simulink model "cap_eq_circuit_pascal5_single_shot_stack"  (R2016b)
settings: Solver=FixedStepAuto  StartTime=0.0  StopTime=sim_time  FixedStep=sim_time*resolution  MinStep=0.001  RelTol=1e-4  EnableMultiTasking=on
values from neighbouring files (symbols this model uses):
  amps_in = double(amps_in)    [Sc.m]    (also in sc_model_single_shot_stack.m; test.m = 0; workspace_nedc_basic_sc.mat = 0; workspace_test_model.mat = 0)
undefined symbols (not defined in the file): capacitance, v_init1, v_init2
libraries: powerlib x360, simulink x8
(part 1 of 5)
settings Model: Creator=ttsh  LastModifiedBy=ttsh
settings SolverCC: ZeroCrossAlgorithm=Adaptive  AlgebraicLoopSolver=LineSearch  SolverResetMethod=Robust
settings DataIOCC: LimitDataPoints=on  SaveFormat=Array
settings OptimizationCC: LifeSpan=inf
settings DebuggingCC: SolverPrmCheckMsg=warning  AllowSymbolicDim=off  SFUnexpectedBacktrackingDiag=warning  SFNoUnconditionalDefaultTransitionDiag=warning  SFExecutionAtInitializationDiag=none
settings HardwareCC: ProdBitPerPointer=32  ProdBitPerSizeT=32  ProdBitPerPtrDiffT=32  ProdLargestAtomicFloat=None  ProdIntDivRoundTo=Undefined  ProdEndianess=Unspecified  ProdWordSize=32  ProdHWDeviceType=32-bit Generic
settings ModelReferenceCC: PropagateSignalLabelsOutOfModel=off
settings GRTTargetCC: TargetLangStandard=C89/C90 (ANSI)  GeneratePreprocessorConditionals=Disable all
settings ConfigComp: CovMetricSettings=dw  CovHtmlReporting=on  CovSaveCumulativeToWorkspaceVar=on  CovSaveSingleToWorkspaceVar=on  CovExternalEMLEnable=off  CovSFcnEnable=off

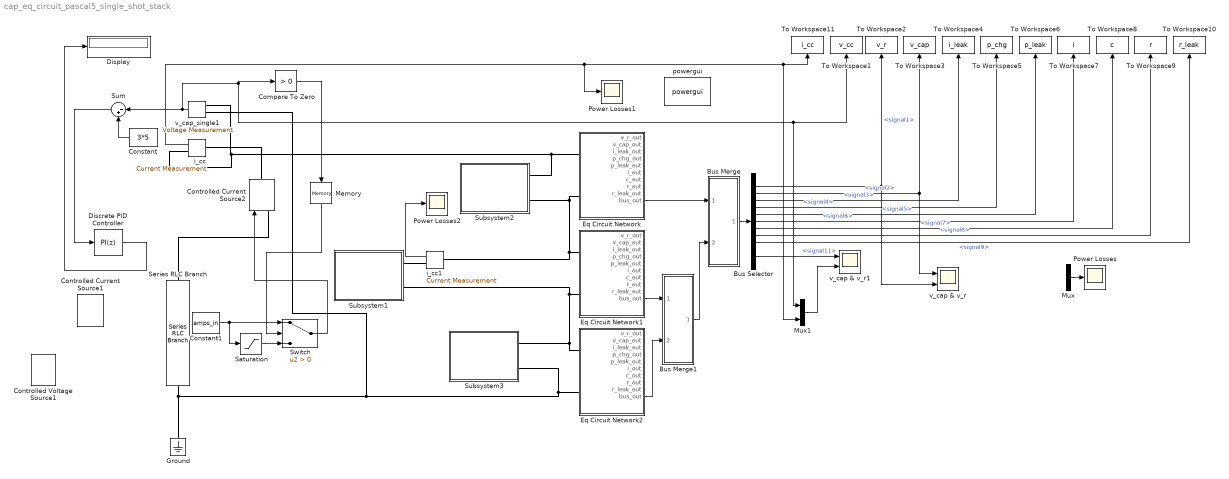
== system cap_eq_circuit_pascal5_single_shot_stack ==
  Bus Selector : BusSelector  OutputSignals=signal1,signal2,signal3,signal4,signal5,signal6,signal7,signal8,signal9,signal10,signal11
  Bus Merge : Subsystem
  Bus Merge1 : Subsystem
  Compare To Zero : simulink/Logic and Bit Operations/Compare To Zero  relop=>  OutDataTypeStr=boolean
  Constant : Constant  Value=3*5
  Constant1 : Constant  Value=amps_in
  Controlled Current Source1 : powerlib/Electrical Sources/Controlled Current Source  Initialize=on  Source_Type=DC  Amplitude=0  Phase=0  Frequency=0  Measurements=None
  Controlled Current Source2 : powerlib/Electrical Sources/Controlled Current Source  Initialize=on  Source_Type=DC  Amplitude=0  Phase=0  Frequency=0  Measurements=None
  Controlled Voltage Source1 : powerlib/Electrical Sources/Controlled Voltage Source  Initialize=on  Source_Type=DC  Amplitude=0  Phase=0  Frequency=0  Measurements=None
  Discrete PID Controller : simulink/Continuous/PID Controller  Controller=PI  TimeDomain=Discrete-time  SampleTime=-1  IntegratorMethod=Forward Euler  FilterMethod=Forward Euler  Form=Parallel  UseFilter=on  ControllerParametersSource=internal  P=1  I=0.02  D=0  N=100  InitialConditionSource=internal  InitialConditionForIntegrator=0  InitialConditionForFilter=0  ExternalReset=none  LimitOutput=on  UpperSaturationLimit=0.1  LowerSaturationLimit=0  LinearizeAsGain=off  AntiWindupMode=none  Kb=1  TrackingMode=off  Kt=1  PParamMin=[]  PParamMax=[]  IParamMin=[]  IParamMax=[]  DParamMin=[]  DParamMax=[]  NParamMin=[]  NParamMax=[]  KbParamMin=[]  KbParamMax=[]  KtParamMin=[]  KtParamMax=[]  POutMin=[]  POutMax=[]  IOutMin=[]  IOutMax=[]  DOutMin=[]  DOutMax=[]  NOutMin=[]  NOutMax=[]  KbOutMin=[]  KbOutMax=[]  KtOutMin=[]  KtOutMax=[]  IntegratorOutMin=[]  IntegratorOutMax=[]  FilterOutMin=[]  FilterOutMax=[]  SumOutMin=[]  SumOutMax=[]  SumI1OutMin=[]  SumI1OutMax=[]  SumI2OutMin=[]  SumI2OutMax=[]  SumI3OutMin=[]  SumI3OutMax=[]  SumDOutMin=[]  SumDOutMax=[]  SaturationOutMin=[]  SaturationOutMax=[]  IntegratorContinuousStateAttributes=''  IntegratorStateMustResolveToSignalObject=off  IntegratorRTWStateStorageClass=Auto  FilterContinuousStateAttributes=''  FilterStateMustResolveToSignalObject=off  FilterRTWStateStorageClass=Auto  DifferentiatorICPrevScaledInput=0  DifferentiatorOutMin=[]  DifferentiatorOutMax=[]
  Display : Display
  Eq Circuit Network : Subsystem  mask{r_leak=inf, c=capacitance, r_esr=0.01, ord=5, v_init1=v_init1(1), v_init2=v_init1(2), v_init3=v_init1(3), v_init4=v_init1(4), v_init5=v_init1(5)}
      mask prompts: r_leak "R Leak /ohm (inf for disabled)"; c "Capacitance /F"; r_esr "ESR"; ord "Elements (pascal order)"; v_init1 "Initial capacitor voltage"; v_init2 "Initial capacitor voltage"; v_init3 "Initial capacitor voltage"; v_init4 "Initial capacitor voltage"; v_init5 "Initial capacitor voltage"
  Eq Circuit Network1 : Subsystem  mask{r_leak=inf, c=capacitance, r_esr=0.01, ord=5, v_init1=v_init2(1), v_init2=v_init2(2), v_init3=v_init2(3), v_init4=v_init2(4), v_init5=v_init2(5)}
      mask prompts: r_leak "R Leak /ohm (inf for disabled)"; c "Capacitance /F"; r_esr "ESR"; ord "Elements (pascal order)"; v_init1 "Initial capacitor voltage"; v_init2 "Initial capacitor voltage"; v_init3 "Initial capacitor voltage"; v_init4 "Initial capacitor voltage"; v_init5 "Initial capacitor voltage"
  Eq Circuit Network2 : Subsystem  mask{r_leak=inf, c=capacitance, r_esr=0.01, ord=5, v_init1=v_init2(1), v_init2=v_init2(2), v_init3=v_init2(3), v_init4=v_init2(4), v_init5=v_init2(5)}
      mask prompts: r_leak "R Leak /ohm (inf for disabled)"; c "Capacitance /F"; r_esr "ESR"; ord "Elements (pascal order)"; v_init1 "Initial capacitor voltage"; v_init2 "Initial capacitor voltage"; v_init3 "Initial capacitor voltage"; v_init4 "Initial capacitor voltage"; v_init5 "Initial capacitor voltage"
  Ground : powerlib/Elements/Ground  LConnTagsString=a
  Memory : Memory  X0=1  InheritSampleTime=on
  Mux : Mux  Inputs=2
  Mux1 : Mux  Inputs=2
  Power Losses : Scope
  Power Losses1 : Scope
  Power Losses2 : Scope
  Saturation : Saturate  UpperLimit=inf  LowerLimit=0
  Series RLC Branch : powerlib/Elements/Series RLC Branch  LConnTagsString=__new0  RConnTagsString=__new0  BranchType=R  Resistance=0.1  Inductance=1e-9  SetiL0=off  InitialCurrent=0  Capacitance=1e-6  Setx0=off  InitialVoltage=0  Measurements=None
  Subsystem1 : Subsystem  mask{r=10, d=0.01, v_cut=5.1, v_min=0}
      mask prompts: r "Series resistance"; d "Rate limit"; v_cut "v cutoff"; v_min "v min"
  Subsystem2 : Subsystem  mask{r=10, d=0.01, v_cut=5.1, v_min=0}
      mask prompts: r "Series resistance"; d "Rate limit"; v_cut "v cutoff"; v_min "v min"
  Subsystem3 : Subsystem  mask{r=10, d=0.01, v_cut=5.1, v_min=0}
      mask prompts: r "Series resistance"; d "Rate limit"; v_cut "v cutoff"; v_min "v min"
  Sum : Sum  Inputs=|-+
  Switch : Switch  Criteria=u2 > Threshold
  To Workspace1 : ToWorkspace  VariableName=v_cc  SampleTime=-1
      settings: Save2DSignal=2-D array (concatenate along first dimension)
  To Workspace10 : ToWorkspace  VariableName=r_leak  SampleTime=-1
      settings: Save2DSignal=2-D array (concatenate along first dimension)
  To Workspace11 : ToWorkspace  VariableName=i_cc  SampleTime=-1
      settings: Save2DSignal=2-D array (concatenate along first dimension)
  To Workspace2 : ToWorkspace  VariableName=v_r  SampleTime=-1
      settings: Save2DSignal=2-D array (concatenate along first dimension)
  To Workspace3 : ToWorkspace  VariableName=v_cap  SampleTime=-1
      settings: Save2DSignal=2-D array (concatenate along first dimension)
  To Workspace4 : ToWorkspace  VariableName=i_leak  SampleTime=-1
      settings: Save2DSignal=2-D array (concatenate along first dimension)
  To Workspace5 : ToWorkspace  VariableName=p_chg  SampleTime=-1
      settings: Save2DSignal=2-D array (concatenate along first dimension)
  To Workspace6 : ToWorkspace  VariableName=p_leak  SampleTime=-1
      settings: Save2DSignal=2-D array (concatenate along first dimension)
  To Workspace7 : ToWorkspace  VariableName=i  SampleTime=-1
      settings: Save2DSignal=2-D array (concatenate along first dimension)
  To Workspace8 : ToWorkspace  VariableName=c  SampleTime=-1
      settings: Save2DSignal=2-D array (concatenate along first dimension)
  To Workspace9 : ToWorkspace  VariableName=r  SampleTime=-1
      settings: Save2DSignal=2-D array (concatenate along first dimension)
  i_cc : powerlib/Measurements/Current Measurement  PhasorSimulation=off  OutputType=Complex  PSBequivalent=0
  i_cc1 : powerlib/Measurements/Current Measurement  PhasorSimulation=off  OutputType=Complex  PSBequivalent=0
  powergui : powerlib/powergui  Priority=1  SimulationMode=Continuous  SolverType=Tustin  SampleTime=50e-6  frequency=60  SPID=on  DisableSnubberDevices=on  DisableRonSwitches=on  DisableVfSwitches=on  SwTol=0  DisplayEquations=off  Interpol=off  ExternalGateDelay=off  methode=off  Ts=0  FunctionMessages=off  echomessages=off  HookPort=off  EnableUseOfTLC=off  x0status=blocks  frequencyindice=0  Pbase=100e6  ErrMax=1e-4  Iterations=50  UnitsV=V  UnitsW=W  buscounter=0  RestoreLinks=warning  ResistiveCurrentMeasurement=off  Frange=[0:2:500]  Ylog=off  Xlog=on  ShowGrid=off  save=off  variable=ZData  structure=0  ZoomFFT=off  StartTime=0.0  cycles=1  DisplayStyle=1  fundamental=60  FreqAxis=off  MaxFrequency=1000  frequencyindicesteady=1  RmsSteady=1  display=off
  v_cap & v_r : Scope  NumInputPorts=2
  v_cap & v_r1 : Scope  NumInputPorts=2
  v_cap_single1 : powerlib/Measurements/Voltage Measurement  PhasorSimulation=off  OutputType=Complex  PSBequivalent=0
  wires:
  Mux/1 -> Power Losses/1
  i_cc/1 -> Power Losses1/1, Mux1/2, To Workspace11/1
  Eq Circuit Network/10(bus_out) -> Bus Merge/1(bus_1_in)
  Bus Merge/1(bus_out) -> Bus Selector/1
  Bus Selector/1 -> v_cap & v_r/2, To Workspace2/1  "<signal1>"
  Bus Selector/2 -> v_cap & v_r/1, To Workspace3/1  "<signal2>"
  Bus Selector/3 -> To Workspace4/1  "<signal3>"
  Bus Selector/4 -> To Workspace5/1  "<signal4>"
  Bus Selector/5 -> To Workspace6/1  "<signal5>"
  Bus Selector/6 -> To Workspace7/1  "<signal6>"
  Bus Selector/7 -> To Workspace8/1  "<signal7>"
  Bus Selector/8 -> To Workspace9/1  "<signal8>"
  Bus Selector/9 -> To Workspace10/1  "<signal9>"
  Bus Selector/11 -> v_cap & v_r1/1  "<signal11>"
  v_cap_single1/1 -> Sum/1, Compare To Zero/1, Mux1/1, To Workspace1/1
  Discrete PID Controller/1 -> Display/1
  Constant/1 -> Sum/2
  Sum/1 -> Discrete PID Controller/1
  Eq Circuit Network1/10(bus_out) -> Bus Merge1/1(bus_1_in)
  Eq Circuit Network2/10(bus_out) -> Bus Merge1/2(bus_2_in)
  Bus Merge1/1(bus_out) -> Bus Merge/2(bus_2_in)
  Mux1/1 -> v_cap & v_r1/2
  i_cc1/1 -> Power Losses2/1
  Constant1/1 -> Switch/1, Saturation/1
  Saturation/1 -> Switch/3
  Compare To Zero/1 -> Memory/1
  Switch/1 -> Controlled Current Source2/1
  Memory/1 -> Switch/2
  connections:
  v_cap_single1/LConn1 -- i_cc/RConn1 -- Subsystem2/RConn1 -- Eq Circuit Network/LConn1
  Eq Circuit Network/LConn2 -- Subsystem2/RConn2 -- i_cc1/LConn1 -- Eq Circuit Network1/LConn1
  Eq Circuit Network1/LConn2 -- Subsystem1/RConn2 -- Eq Circuit Network2/LConn1 -- Subsystem3/RConn1
  Controlled Current Source2/LConn1 -- Series RLC Branch/LConn1
  Controlled Current Source2/RConn1 -- i_cc/LConn1
  Series RLC Branch/RConn1 -- Ground/LConn1 -- v_cap_single1/LConn2 -- Eq Circuit Network2/LConn2 -- Subsystem3/RConn2
  Subsystem1/RConn1 -- i_cc1/RConn1

== system cap_eq_circuit_pascal5_single_shot_stack/Bus Merge ==
  bus_1_in : Inport
  bus_2_in : Inport  Port=2
  Bus Creator : BusCreator  Inputs=11
  Bus Selector : BusSelector  OutputSignals=signal1,signal2,signal3,signal4,signal5,signal6,signal7,signal8,signal9,signal10,signal11
  Bus Selector1 : BusSelector  OutputSignals=signal1,signal2,signal3,signal4,signal5,signal6,signal7,signal8,signal9,signal10,signal11
  Mux{1..11} (11 alike) : Mux  Inputs=2
  bus_out : Outport
  wires:
  bus_1_in/1 -> Bus Selector/1
  bus_2_in/1 -> Bus Selector1/1
  Bus Creator/1 -> bus_out/1
  Bus Selector/1 -> Mux1/1  "<signal1>"
  Bus Selector1/2 -> Mux2/2  "<signal2>"
  Bus Selector/3 -> Mux3/1  "<signal3>"
  Bus Selector1/4 -> Mux4/2  "<signal4>"
  Bus Selector/5 -> Mux5/1  "<signal5>"
  Bus Selector1/6 -> Mux6/1  "<signal6>"
  Bus Selector/7 -> Mux7/1  "<signal7>"
  Bus Selector1/8 -> Mux8/1  "<signal8>"
  Bus Selector1/10 -> Mux10/1  "<signal10>"
  Bus Selector/11 -> Mux11/1  "<signal11>"
  Bus Selector/9 -> Mux9/1  "<signal9>"
  Bus Selector/2 -> Mux2/1  "<signal2>"
  Bus Selector/4 -> Mux4/1  "<signal4>"
  Bus Selector/6 -> Mux6/2  "<signal6>"
  Bus Selector/8 -> Mux8/2  "<signal8>"
  Bus Selector/10 -> Mux10/2  "<signal10>"
  Bus Selector1/1 -> Mux1/2  "<signal1>"
  Bus Selector1/3 -> Mux3/2  "<signal3>"
  Bus Selector1/5 -> Mux5/2  "<signal5>"
  Bus Selector1/7 -> Mux7/2  "<signal7>"
  Bus Selector1/9 -> Mux9/2  "<signal9>"
  Bus Selector1/11 -> Mux11/2  "<signal11>"
  Mux1/1 -> Bus Creator/1
  Mux3/1 -> Bus Creator/3
  Mux5/1 -> Bus Creator/5
  Mux7/1 -> Bus Creator/7
  Mux9/1 -> Bus Creator/9
  Mux11/1 -> Bus Creator/11
  Mux2/1 -> Bus Creator/2
  Mux4/1 -> Bus Creator/4
  Mux6/1 -> Bus Creator/6
  Mux8/1 -> Bus Creator/8
  Mux10/1 -> Bus Creator/10

== system cap_eq_circuit_pascal5_single_shot_stack/Bus Merge1 ==
  bus_1_in : Inport
  bus_2_in : Inport  Port=2
  Bus Creator : BusCreator  Inputs=11
  Bus Selector : BusSelector  OutputSignals=signal1,signal2,signal3,signal4,signal5,signal6,signal7,signal8,signal9,signal10,signal11
  Bus Selector1 : BusSelector  OutputSignals=signal1,signal2,signal3,signal4,signal5,signal6,signal7,signal8,signal9,signal10,signal11
  Mux{1..11} (11 alike) : Mux  Inputs=2
  bus_out : Outport
  wires:
  Mux10/1 -> Bus Creator/10
  Mux8/1 -> Bus Creator/8
  Mux6/1 -> Bus Creator/6
  Mux4/1 -> Bus Creator/4
  Mux2/1 -> Bus Creator/2
  Mux11/1 -> Bus Creator/11
  Mux9/1 -> Bus Creator/9
  Mux7/1 -> Bus Creator/7
  Mux5/1 -> Bus Creator/5
  Mux3/1 -> Bus Creator/3
  Mux1/1 -> Bus Creator/1
  Bus Selector1/11 -> Mux11/2  "<signal11>"
  Bus Selector1/9 -> Mux9/2  "<signal9>"
  Bus Selector1/7 -> Mux7/2  "<signal7>"
  Bus Selector1/5 -> Mux5/2  "<signal5>"
  Bus Selector1/3 -> Mux3/2  "<signal3>"
  Bus Selector1/1 -> Mux1/2  "<signal1>"
  Bus Selector/10 -> Mux10/2  "<signal10>"
  Bus Selector/8 -> Mux8/2  "<signal8>"
  Bus Selector/6 -> Mux6/2  "<signal6>"
  Bus Selector/4 -> Mux4/1  "<signal4>"
  Bus Selector/2 -> Mux2/1  "<signal2>"
  Bus Selector/9 -> Mux9/1  "<signal9>"
  Bus Selector/11 -> Mux11/1  "<signal11>"
  Bus Selector1/10 -> Mux10/1  "<signal10>"
  Bus Selector1/8 -> Mux8/1  "<signal8>"
  Bus Selector/7 -> Mux7/1  "<signal7>"
  Bus Selector1/6 -> Mux6/1  "<signal6>"
  Bus Selector/5 -> Mux5/1  "<signal5>"
  Bus Selector1/4 -> Mux4/2  "<signal4>"
  Bus Selector/3 -> Mux3/1  "<signal3>"
  Bus Selector1/2 -> Mux2/2  "<signal2>"
  Bus Selector/1 -> Mux1/1  "<signal1>"
  Bus Creator/1 -> bus_out/1
  bus_2_in/1 -> Bus Selector1/1
  bus_1_in/1 -> Bus Selector/1

== system cap_eq_circuit_pascal5_single_shot_stack/Eq Circuit Network ==
  note: 6x 700R
  note: 4x 1k4
  note: 4x 625R
  note: 1x 550R
  note: 1x 4k
  Bus Creator : BusCreator  Inputs=11
  Subsystem : Subsystem  mask{c=c, r_esr=625, r_leak=r_leak, v_init=v_init2}
      mask prompts: c "Capacitance /F"; r_esr "Series resistance /ohm"; r_leak "Leak resistance /ohm (inf for disabled)"; v_init "Initial capacitor voltage"
  Subsystem1 : Subsystem  mask{c=c, r_esr=1.4e3, r_leak=r_leak, v_init=v_init4}
      mask prompts: c "Capacitance /F"; r_esr "Series resistance /ohm"; r_leak "Leak resistance /ohm (inf for disabled)"; v_init "Initial capacitor voltage"
  Subsystem2 : Subsystem  mask{c=c, r_esr=700, r_leak=r_leak, v_init=v_init3}
      mask prompts: c "Capacitance /F"; r_esr "Series resistance /ohm"; r_leak "Leak resistance /ohm (inf for disabled)"; v_init "Initial capacitor voltage"
  Subsystem5 : Subsystem  mask{c=c, r_esr=4e3, r_leak=r_leak, v_init=v_init5}
      mask prompts: c "Capacitance /F"; r_esr "Series resistance /ohm"; r_leak "Leakage resistance /ohm (inf for disabled)"; v_init "Initial capacitor voltage"
  Subsystem8 : Subsystem  mask{c=c, r_esr=550, r_leak=r_leak, v_init=v_init1}
      mask prompts: c "Capacitance /F"; r_esr "Series resistance /ohm"; r_leak "Leakage resistance /ohm (inf for disabled)"; v_init "Initial capacitor voltage"
  v_cap_single : powerlib/Measurements/Voltage Measurement  PhasorSimulation=off  OutputType=Complex  PSBequivalent=0
  VCC_in : PMIOPort  Port=1  Side=Left
  VSS_in : PMIOPort  Port=2  Side=Left
  VCC_out : PMIOPort  Port=3  Side=Right
  VSS_out : PMIOPort  Port=4  Side=Right
  v_r_out : Outport
  v_cap_out : Outport  Port=2
  i_leak_out : Outport  Port=3
  p_chg_out : Outport  Port=4
  p_leak_out : Outport  Port=5
  i_out : Outport  Port=6
  c_out : Outport  Port=7
  r_out : Outport  Port=8
  r_leak_out : Outport  Port=9
  bus_out : Outport  Port=10
  wires:
  Subsystem5/5(p_leak_out) -> Bus Creator/5, p_leak_out/1
  Subsystem5/6(i_out) -> Bus Creator/6, i_out/1
  Subsystem5/4(p_chg_out) -> Bus Creator/4, p_chg_out/1
  Subsystem5/7(c_out) -> Bus Creator/7, c_out/1
  Subsystem5/3(i_leak_out) -> Bus Creator/3, i_leak_out/1
  Subsystem5/8(r_out) -> Bus Creator/8, r_out/1
  Subsystem5/2(v_cap_out) -> Bus Creator/2, v_cap_out/1
  Subsystem5/9(r_leak_out) -> Bus Creator/9, r_leak_out/1
  Subsystem5/1(v_r_out) -> Bus Creator/1, v_r_out/1
  Subsystem8/3(i_leak_out) -> Subsystem/3(In3)
  Subsystem8/6(i_out) -> Subsystem/6(In6)
  Subsystem8/9(r_leak_out) -> Subsystem/9(In9)
  Subsystem8/4(p_chg_out) -> Subsystem/4(In4)
  Subsystem8/10(l_out) -> Subsystem/10(In10)
  Subsystem8/8(r_out) -> Subsystem/8(In8)
  Subsystem8/5(p_leak_out) -> Subsystem/5(In5)
  Subsystem8/7(c_out) -> Subsystem/7(In7)
  Subsystem8/1(v_r_out) -> Subsystem/1(In1)
  Subsystem8/2(v_cap_out) -> Subsystem/2(In2)
  Subsystem1/6(Out6) -> Subsystem5/6(i_in)
  Subsystem1/8(Out8) -> Subsystem5/8(r_in)
  Subsystem1/4(Out4) -> Subsystem5/4(p_chg_in)
  Subsystem1/7(Out7) -> Subsystem5/7(c_in)
  Subsystem1/9(Out9) -> Subsystem5/9(r_leak_in)
  Subsystem1/3(Out3) -> Subsystem5/3(i_leak_in)
  Subsystem1/10(Out10) -> Subsystem5/10(l_in)
  Subsystem1/5(Out5) -> Subsystem5/5(p_leak_in)
  Subsystem1/2(Out2) -> Subsystem5/2(v_cap_in)
  Subsystem1/1(Out1) -> Subsystem5/1(v_r_in)
  Subsystem/3(Out3) -> Subsystem2/3(In3)
  Subsystem/10(Out10) -> Subsystem2/10(In10)
  Subsystem/8(Out8) -> Subsystem2/8(In8)
  Subsystem/1(Out1) -> Subsystem2/1(In1)
  Subsystem/2(Out2) -> Subsystem2/2(In2)
  Subsystem/6(Out6) -> Subsystem2/6(In6)
  Subsystem/9(Out9) -> Subsystem2/9(In9)
  Subsystem/7(Out7) -> Subsystem2/7(In7)
  Subsystem/4(Out4) -> Subsystem2/4(In4)
  Subsystem/5(Out5) -> Subsystem2/5(In5)
  Subsystem2/5(Out5) -> Subsystem1/5(In5)
  Subsystem2/8(Out8) -> Subsystem1/8(In8)
  Subsystem2/6(Out6) -> Subsystem1/6(In6)
  Subsystem2/2(Out2) -> Subsystem1/2(In2)
  Subsystem2/10(Out10) -> Subsystem1/10(In10)
  Subsystem2/9(Out9) -> Subsystem1/9(In9)
  Subsystem2/1(Out1) -> Subsystem1/1(In1)
  Subsystem2/3(Out3) -> Subsystem1/3(In3)
  Subsystem2/4(Out4) -> Subsystem1/4(In4)
  Subsystem2/7(Out7) -> Subsystem1/7(In7)
  v_cap_single/1 -> Bus Creator/11
  Subsystem5/10(l_out) -> Bus Creator/10
  Bus Creator/1 -> bus_out/1
  connections:
  Subsystem8/LConn1 -- VCC_in/RConn1
  VSS_in/RConn1 -- Subsystem8/LConn2
  Subsystem8/RConn2 -- Subsystem/LConn2
  Subsystem8/RConn1 -- Subsystem/LConn1
  Subsystem1/RConn2 -- Subsystem5/LConn2
  Subsystem1/RConn1 -- Subsystem5/LConn1
  Subsystem/RConn1 -- Subsystem2/LConn1
  Subsystem/RConn2 -- Subsystem2/LConn2
  Subsystem1/LConn2 -- Subsystem2/RConn2
  Subsystem1/LConn1 -- Subsystem2/RConn1
  VCC_out/RConn1 -- v_cap_single/LConn1 -- Subsystem5/RConn1
  Subsystem5/RConn2 -- v_cap_single/LConn2 -- VSS_out/RConn1

== system cap_eq_circuit_pascal5_single_shot_stack/Eq Circuit Network1 ==
  note: 1x 4k
  note: 1x 550R
  note: 4x 625R
  note: 4x 1k4
  note: 6x 700R
  Bus Creator : BusCreator  Inputs=11
  Subsystem : Subsystem  mask{c=c, r_esr=625, r_leak=r_leak, v_init=v_init2}
      mask prompts: c "Capacitance /F"; r_esr "Series resistance /ohm"; r_leak "Leak resistance /ohm (inf for disabled)"; v_init "Initial capacitor voltage"
  Subsystem1 : Subsystem  mask{c=c, r_esr=1.4e3, r_leak=r_leak, v_init=v_init4}
      mask prompts: c "Capacitance /F"; r_esr "Series resistance /ohm"; r_leak "Leak resistance /ohm (inf for disabled)"; v_init "Initial capacitor voltage"
  Subsystem2 : Subsystem  mask{c=c, r_esr=700, r_leak=r_leak, v_init=v_init3}
      mask prompts: c "Capacitance /F"; r_esr "Series resistance /ohm"; r_leak "Leak resistance /ohm (inf for disabled)"; v_init "Initial capacitor voltage"
  Subsystem5 : Subsystem  mask{c=c, r_esr=4e3, r_leak=r_leak, v_init=v_init5}
      mask prompts: c "Capacitance /F"; r_esr "Series resistance /ohm"; r_leak "Leakage resistance /ohm (inf for disabled)"; v_init "Initial capacitor voltage"
  Subsystem8 : Subsystem  mask{c=c, r_esr=550, r_leak=r_leak, v_init=v_init1}
      mask prompts: c "Capacitance /F"; r_esr "Series resistance /ohm"; r_leak "Leakage resistance /ohm (inf for disabled)"; v_init "Initial capacitor voltage"
  v_cap_single : powerlib/Measurements/Voltage Measurement  PhasorSimulation=off  OutputType=Complex  PSBequivalent=0
  VCC_in : PMIOPort  Port=1  Side=Left
  VSS_in : PMIOPort  Port=2  Side=Left
  VCC_out : PMIOPort  Port=3  Side=Right
  VSS_out : PMIOPort  Port=4  Side=Right
  v_r_out : Outport
  v_cap_out : Outport  Port=2
  i_leak_out : Outport  Port=3
  p_chg_out : Outport  Port=4
  p_leak_out : Outport  Port=5
  i_out : Outport  Port=6
  c_out : Outport  Port=7
  r_out : Outport  Port=8
  r_leak_out : Outport  Port=9
  bus_out : Outport  Port=10
  wires:
  Bus Creator/1 -> bus_out/1
  Subsystem5/10(l_out) -> Bus Creator/10
  v_cap_single/1 -> Bus Creator/11
  Subsystem2/7(Out7) -> Subsystem1/7(In7)
  Subsystem2/4(Out4) -> Subsystem1/4(In4)
  Subsystem2/3(Out3) -> Subsystem1/3(In3)
  Subsystem2/1(Out1) -> Subsystem1/1(In1)
  Subsystem2/9(Out9) -> Subsystem1/9(In9)
  Subsystem2/10(Out10) -> Subsystem1/10(In10)
  Subsystem2/2(Out2) -> Subsystem1/2(In2)
  Subsystem2/6(Out6) -> Subsystem1/6(In6)
  Subsystem2/8(Out8) -> Subsystem1/8(In8)
  Subsystem2/5(Out5) -> Subsystem1/5(In5)
  Subsystem/5(Out5) -> Subsystem2/5(In5)
  Subsystem/4(Out4) -> Subsystem2/4(In4)
  Subsystem/7(Out7) -> Subsystem2/7(In7)
  Subsystem/9(Out9) -> Subsystem2/9(In9)
  Subsystem/6(Out6) -> Subsystem2/6(In6)
  Subsystem/2(Out2) -> Subsystem2/2(In2)
  Subsystem/1(Out1) -> Subsystem2/1(In1)
  Subsystem/8(Out8) -> Subsystem2/8(In8)
  Subsystem/10(Out10) -> Subsystem2/10(In10)
  Subsystem/3(Out3) -> Subsystem2/3(In3)
  Subsystem1/1(Out1) -> Subsystem5/1(v_r_in)
  Subsystem1/2(Out2) -> Subsystem5/2(v_cap_in)
  Subsystem1/5(Out5) -> Subsystem5/5(p_leak_in)
  Subsystem1/10(Out10) -> Subsystem5/10(l_in)
  Subsystem1/3(Out3) -> Subsystem5/3(i_leak_in)
  Subsystem1/9(Out9) -> Subsystem5/9(r_leak_in)
  Subsystem1/7(Out7) -> Subsystem5/7(c_in)
  Subsystem1/4(Out4) -> Subsystem5/4(p_chg_in)
  Subsystem1/8(Out8) -> Subsystem5/8(r_in)
  Subsystem1/6(Out6) -> Subsystem5/6(i_in)
  Subsystem8/2(v_cap_out) -> Subsystem/2(In2)
  Subsystem8/1(v_r_out) -> Subsystem/1(In1)
  Subsystem8/7(c_out) -> Subsystem/7(In7)
  Subsystem8/5(p_leak_out) -> Subsystem/5(In5)
  Subsystem8/8(r_out) -> Subsystem/8(In8)
  Subsystem8/10(l_out) -> Subsystem/10(In10)
  Subsystem8/4(p_chg_out) -> Subsystem/4(In4)
  Subsystem8/9(r_leak_out) -> Subsystem/9(In9)
  Subsystem8/6(i_out) -> Subsystem/6(In6)
  Subsystem8/3(i_leak_out) -> Subsystem/3(In3)
  Subsystem5/1(v_r_out) -> v_r_out/1, Bus Creator/1
  Subsystem5/9(r_leak_out) -> r_leak_out/1, Bus Creator/9
  Subsystem5/2(v_cap_out) -> v_cap_out/1, Bus Creator/2
  Subsystem5/8(r_out) -> r_out/1, Bus Creator/8
  Subsystem5/3(i_leak_out) -> i_leak_out/1, Bus Creator/3
  Subsystem5/7(c_out) -> c_out/1, Bus Creator/7
  Subsystem5/4(p_chg_out) -> p_chg_out/1, Bus Creator/4
  Subsystem5/6(i_out) -> i_out/1, Bus Creator/6
  Subsystem5/5(p_leak_out) -> p_leak_out/1, Bus Creator/5
  connections:
  v_cap_single/LConn2 -- Subsystem5/RConn2 -- VSS_out/RConn1
  v_cap_single/LConn1 -- VCC_out/RConn1 -- Subsystem5/RConn1
  Subsystem1/LConn1 -- Subsystem2/RConn1
  Subsystem1/LConn2 -- Subsystem2/RConn2
  Subsystem/RConn2 -- Subsystem2/LConn2
  Subsystem/RConn1 -- Subsystem2/LConn1
  Subsystem1/RConn1 -- Subsystem5/LConn1
  Subsystem1/RConn2 -- Subsystem5/LConn2
  Subsystem8/RConn1 -- Subsystem/LConn1
  Subsystem8/RConn2 -- Subsystem/LConn2
  VSS_in/RConn1 -- Subsystem8/LConn2
  Subsystem8/LConn1 -- VCC_in/RConn1

== system cap_eq_circuit_pascal5_single_shot_stack/Eq Circuit Network2 ==
  note: 6x 700R
  note: 4x 1k4
  note: 4x 625R
  note: 1x 550R
  note: 1x 4k
  Bus Creator : BusCreator  Inputs=11
  Subsystem : Subsystem  mask{c=c, r_esr=625, r_leak=r_leak, v_init=v_init2}
      mask prompts: c "Capacitance /F"; r_esr "Series resistance /ohm"; r_leak "Leak resistance /ohm (inf for disabled)"; v_init "Initial capacitor voltage"
  Subsystem1 : Subsystem  mask{c=c, r_esr=1.4e3, r_leak=r_leak, v_init=v_init4}
      mask prompts: c "Capacitance /F"; r_esr "Series resistance /ohm"; r_leak "Leak resistance /ohm (inf for disabled)"; v_init "Initial capacitor voltage"
  Subsystem2 : Subsystem  mask{c=c, r_esr=700, r_leak=r_leak, v_init=v_init3}
      mask prompts: c "Capacitance /F"; r_esr "Series resistance /ohm"; r_leak "Leak resistance /ohm (inf for disabled)"; v_init "Initial capacitor voltage"
  Subsystem5 : Subsystem  mask{c=c, r_esr=4e3, r_leak=r_leak, v_init=v_init5}
      mask prompts: c "Capacitance /F"; r_esr "Series resistance /ohm"; r_leak "Leakage resistance /ohm (inf for disabled)"; v_init "Initial capacitor voltage"
  Subsystem8 : Subsystem  mask{c=c, r_esr=550, r_leak=r_leak, v_init=v_init1}
      mask prompts: c "Capacitance /F"; r_esr "Series resistance /ohm"; r_leak "Leakage resistance /ohm (inf for disabled)"; v_init "Initial capacitor voltage"
  v_cap_single : powerlib/Measurements/Voltage Measurement  PhasorSimulation=off  OutputType=Complex  PSBequivalent=0
  VCC_in : PMIOPort  Port=1  Side=Left
  VSS_in : PMIOPort  Port=2  Side=Left
  VCC_out : PMIOPort  Port=3  Side=Right
  VSS_out : PMIOPort  Port=4  Side=Right
  v_r_out : Outport
  v_cap_out : Outport  Port=2
  i_leak_out : Outport  Port=3
  p_chg_out : Outport  Port=4
  p_leak_out : Outport  Port=5
  i_out : Outport  Port=6
  c_out : Outport  Port=7
  r_out : Outport  Port=8
  r_leak_out : Outport  Port=9
  bus_out : Outport  Port=10
  wires:
  Subsystem5/5(p_leak_out) -> Bus Creator/5, p_leak_out/1
  Subsystem5/6(i_out) -> Bus Creator/6, i_out/1
  Subsystem5/4(p_chg_out) -> Bus Creator/4, p_chg_out/1
  Subsystem5/7(c_out) -> Bus Creator/7, c_out/1
  Subsystem5/3(i_leak_out) -> Bus Creator/3, i_leak_out/1
  Subsystem5/8(r_out) -> Bus Creator/8, r_out/1
  Subsystem5/2(v_cap_out) -> Bus Creator/2, v_cap_out/1
  Subsystem5/9(r_leak_out) -> Bus Creator/9, r_leak_out/1
  Subsystem5/1(v_r_out) -> Bus Creator/1, v_r_out/1
  Subsystem8/3(i_leak_out) -> Subsystem/3(In3)
  Subsystem8/6(i_out) -> Subsystem/6(In6)
  Subsystem8/9(r_leak_out) -> Subsystem/9(In9)
  Subsystem8/4(p_chg_out) -> Subsystem/4(In4)
  Subsystem8/10(l_out) -> Subsystem/10(In10)
  Subsystem8/8(r_out) -> Subsystem/8(In8)
  Subsystem8/5(p_leak_out) -> Subsystem/5(In5)
  Subsystem8/7(c_out) -> Subsystem/7(In7)
  Subsystem8/1(v_r_out) -> Subsystem/1(In1)
  Subsystem8/2(v_cap_out) -> Subsystem/2(In2)
  Subsystem1/6(Out6) -> Subsystem5/6(i_in)
  Subsystem1/8(Out8) -> Subsystem5/8(r_in)
  Subsystem1/4(Out4) -> Subsystem5/4(p_chg_in)
  Subsystem1/7(Out7) -> Subsystem5/7(c_in)
  Subsystem1/9(Out9) -> Subsystem5/9(r_leak_in)
  Subsystem1/3(Out3) -> Subsystem5/3(i_leak_in)
  Subsystem1/10(Out10) -> Subsystem5/10(l_in)
  Subsystem1/5(Out5) -> Subsystem5/5(p_leak_in)
  Subsystem1/2(Out2) -> Subsystem5/2(v_cap_in)
  Subsystem1/1(Out1) -> Subsystem5/1(v_r_in)
  Subsystem/3(Out3) -> Subsystem2/3(In3)
  Subsystem/10(Out10) -> Subsystem2/10(In10)
  Subsystem/8(Out8) -> Subsystem2/8(In8)
  Subsystem/1(Out1) -> Subsystem2/1(In1)
  Subsystem/2(Out2) -> Subsystem2/2(In2)
  Subsystem/6(Out6) -> Subsystem2/6(In6)
  Subsystem/9(Out9) -> Subsystem2/9(In9)
  Subsystem/7(Out7) -> Subsystem2/7(In7)
  Subsystem/4(Out4) -> Subsystem2/4(In4)
  Subsystem/5(Out5) -> Subsystem2/5(In5)
  Subsystem2/5(Out5) -> Subsystem1/5(In5)
  Subsystem2/8(Out8) -> Subsystem1/8(In8)
  Subsystem2/6(Out6) -> Subsystem1/6(In6)
  Subsystem2/2(Out2) -> Subsystem1/2(In2)
  Subsystem2/10(Out10) -> Subsystem1/10(In10)
  Subsystem2/9(Out9) -> Subsystem1/9(In9)
  Subsystem2/1(Out1) -> Subsystem1/1(In1)
  Subsystem2/3(Out3) -> Subsystem1/3(In3)
  Subsystem2/4(Out4) -> Subsystem1/4(In4)
  Subsystem2/7(Out7) -> Subsystem1/7(In7)
  v_cap_single/1 -> Bus Creator/11
  Subsystem5/10(l_out) -> Bus Creator/10
  Bus Creator/1 -> bus_out/1
  connections:
  Subsystem8/LConn1 -- VCC_in/RConn1
  VSS_in/RConn1 -- Subsystem8/LConn2
  Subsystem8/RConn2 -- Subsystem/LConn2
  Subsystem8/RConn1 -- Subsystem/LConn1
  Subsystem1/RConn2 -- Subsystem5/LConn2
  Subsystem1/RConn1 -- Subsystem5/LConn1
  Subsystem/RConn1 -- Subsystem2/LConn1
  Subsystem/RConn2 -- Subsystem2/LConn2
  Subsystem1/LConn2 -- Subsystem2/RConn2
  Subsystem1/LConn1 -- Subsystem2/RConn1
  Subsystem5/RConn1 -- VCC_out/RConn1 -- v_cap_single/LConn1
  VSS_out/RConn1 -- Subsystem5/RConn2 -- v_cap_single/LConn2

== system cap_eq_circuit_pascal5_single_shot_stack/Subsystem1 ==
  Compare To Constant : simulink/Logic and Bit Operations/Compare To Constant  relop=>  const=v_cut  OutDataTypeStr=uint8
  Compare To Constant1 : simulink/Logic and Bit Operations/Compare To Constant  relop=<  const=v_min  OutDataTypeStr=uint8
  Gain : Gain  Gain=5  OutDataTypeStr=double
  Gain1 : Gain  Gain=5  OutDataTypeStr=double
  Mosfet : powerlib/Power Electronics/Mosfet  Ron=0.1  Lon=0  Rd=0.01  Vfd=0  IC=0  Rs=1e5  Cs=inf  Measurements=off
  Mosfet1 : powerlib/Power Electronics/Mosfet  Ron=0.1  Lon=0  Rd=0.01  Vfd=0  IC=0  Rs=1e5  Cs=inf  Measurements=off
  Power Losses2 : Scope
  Rate Limiter : RateLimiter  RisingSlewLimit=d  FallingSlewLimit=-d  SampleTimeMode=inherited
  Series RLC Branch1 : powerlib/Elements/Series RLC Branch  LConnTagsString=__new0  RConnTagsString=__new0  BranchType=R  Resistance=r  Inductance=1e-3  SetiL0=off  InitialCurrent=0  Capacitance=1e-6  Setx0=off  InitialVoltage=0  Measurements=None
  Sum : Sum  Inputs=++|
  v_cap_single2 : powerlib/Measurements/Voltage Measurement  PhasorSimulation=off  OutputType=Complex  PSBequivalent=0
  vcc : PMIOPort  Port=1  Side=Right
  vss : PMIOPort  Port=2  Side=Right
  wires:
  Compare To Constant/1 -> Gain/1
  v_cap_single2/1 -> Compare To Constant1/1, Compare To Constant/1
  Sum/1 -> Rate Limiter/1
  Compare To Constant1/1 -> Gain1/1
  Rate Limiter/1 -> Power Losses2/1, Mosfet/1, Mosfet1/1
  Gain/1 -> Sum/2
  Gain1/1 -> Sum/1
  connections:
  Mosfet1/LConn1 -- Mosfet/LConn1
  v_cap_single2/LConn1 -- vcc/RConn1 -- Mosfet1/RConn1
  v_cap_single2/LConn2 -- Series RLC Branch1/RConn1 -- vss/RConn1
  Mosfet/RConn1 -- Series RLC Branch1/LConn1

== system cap_eq_circuit_pascal5_single_shot_stack/Subsystem2 ==
  Compare To Constant : simulink/Logic and Bit Operations/Compare To Constant  relop=>  const=v_cut  OutDataTypeStr=uint8
  Compare To Constant1 : simulink/Logic and Bit Operations/Compare To Constant  relop=<  const=v_min  OutDataTypeStr=uint8
  Gain : Gain  Gain=5  OutDataTypeStr=double
  Gain1 : Gain  Gain=5  OutDataTypeStr=double
  Mosfet : powerlib/Power Electronics/Mosfet  Ron=0.1  Lon=0  Rd=0.01  Vfd=0  IC=0  Rs=1e5  Cs=inf  Measurements=off
  Mosfet1 : powerlib/Power Electronics/Mosfet  Ron=0.1  Lon=0  Rd=0.01  Vfd=0  IC=0  Rs=1e5  Cs=inf  Measurements=off
  Power Losses2 : Scope
  Rate Limiter : RateLimiter  RisingSlewLimit=d  FallingSlewLimit=-d  SampleTimeMode=inherited
  Series RLC Branch1 : powerlib/Elements/Series RLC Branch  LConnTagsString=__new0  RConnTagsString=__new0  BranchType=R  Resistance=r  Inductance=1e-3  SetiL0=off  InitialCurrent=0  Capacitance=1e-6  Setx0=off  InitialVoltage=0  Measurements=None
  Sum : Sum  Inputs=++|
  v_cap_single2 : powerlib/Measurements/Voltage Measurement  PhasorSimulation=off  OutputType=Complex  PSBequivalent=0
  vcc : PMIOPort  Port=1  Side=Right
  vss : PMIOPort  Port=2  Side=Right
  wires:
  Gain1/1 -> Sum/1
  Gain/1 -> Sum/2
  Rate Limiter/1 -> Mosfet1/1, Mosfet/1, Power Losses2/1
  Compare To Constant1/1 -> Gain1/1
  Sum/1 -> Rate Limiter/1
  v_cap_single2/1 -> Compare To Constant/1, Compare To Constant1/1
  Compare To Constant/1 -> Gain/1
  connections:
  Mosfet/RConn1 -- Series RLC Branch1/LConn1
  vss/RConn1 -- Series RLC Branch1/RConn1 -- v_cap_single2/LConn2
  Mosfet1/RConn1 -- vcc/RConn1 -- v_cap_single2/LConn1
  Mosfet1/LConn1 -- Mosfet/LConn1

== system cap_eq_circuit_pascal5_single_shot_stack/Subsystem3 ==
  Compare To Constant : simulink/Logic and Bit Operations/Compare To Constant  relop=>  const=v_cut  OutDataTypeStr=uint8
  Compare To Constant1 : simulink/Logic and Bit Operations/Compare To Constant  relop=<  const=v_min  OutDataTypeStr=uint8
  Gain : Gain  Gain=5  OutDataTypeStr=double
  Gain1 : Gain  Gain=5  OutDataTypeStr=double
  Mosfet : powerlib/Power Electronics/Mosfet  Ron=0.1  Lon=0  Rd=0.01  Vfd=0  IC=0  Rs=1e5  Cs=inf  Measurements=off
  Mosfet1 : powerlib/Power Electronics/Mosfet  Ron=0.1  Lon=0  Rd=0.01  Vfd=0  IC=0  Rs=1e5  Cs=inf  Measurements=off
  Power Losses2 : Scope
  Rate Limiter : RateLimiter  RisingSlewLimit=d  FallingSlewLimit=-d  SampleTimeMode=inherited
  Series RLC Branch1 : powerlib/Elements/Series RLC Branch  LConnTagsString=__new0  RConnTagsString=__new0  BranchType=R  Resistance=r  Inductance=1e-3  SetiL0=off  InitialCurrent=0  Capacitance=1e-6  Setx0=off  InitialVoltage=0  Measurements=None
  Sum : Sum  Inputs=++|
  v_cap_single2 : powerlib/Measurements/Voltage Measurement  PhasorSimulation=off  OutputType=Complex  PSBequivalent=0
  vcc : PMIOPort  Port=1  Side=Right
  vss : PMIOPort  Port=2  Side=Right
  wires:
  Compare To Constant/1 -> Gain/1
  v_cap_single2/1 -> Compare To Constant1/1, Compare To Constant/1
  Sum/1 -> Rate Limiter/1
  Compare To Constant1/1 -> Gain1/1
  Rate Limiter/1 -> Power Losses2/1, Mosfet/1, Mosfet1/1
  Gain/1 -> Sum/2
  Gain1/1 -> Sum/1
  connections:
  Mosfet1/LConn1 -- Mosfet/LConn1
  v_cap_single2/LConn1 -- vcc/RConn1 -- Mosfet1/RConn1
  v_cap_single2/LConn2 -- Series RLC Branch1/RConn1 -- vss/RConn1
  Mosfet/RConn1 -- Series RLC Branch1/LConn1

== system cap_eq_circuit_pascal5_single_shot_stack/Eq Circuit Network/Subsystem ==
  In1 : Inport
  In2 : Inport  Port=2
  In3 : Inport  Port=3
  In4 : Inport  Port=4
  In5 : Inport  Port=5
  In6 : Inport  Port=6
  In7 : Inport  Port=7
  In8 : Inport  Port=8
  In9 : Inport  Port=9
  In10 : Inport  Port=10
  Subsystem1 : Subsystem  mask{c=c, r_esr=r_esr, r_leak=r_leak, v_init=v_init}
      mask prompts: c "Capacitance /F"; r_esr "Series resistance /ohm"; r_leak "Leakage resistance /ohm (inf for disabled)"; v_init "Initial capacitor voltage"
  Subsystem2 : Subsystem  mask{c=c, r_esr=r_esr, r_leak=r_leak, v_init=v_init}
      mask prompts: c "Capacitance /F"; r_esr "Series resistance /ohm"; r_leak "Leakage resistance /ohm (inf for disabled)"; v_init "Initial capacitor voltage"
  Subsystem3 : Subsystem  mask{c=c, r_esr=r_esr, r_leak=r_leak, v_init=v_init}
      mask prompts: c "Capacitance /F"; r_esr "Series resistance /ohm"; r_leak "Leakage resistance /ohm (inf for disabled)"; v_init "Initial capacitor voltage"
  Subsystem5 : Subsystem  mask{c=c, r_esr=r_esr, r_leak=r_leak, v_init=v_init}
      mask prompts: c "Capacitance /F"; r_esr "Series resistance /ohm"; r_leak "Leakage resistance /ohm (inf for disabled)"; v_init "Initial capacitor voltage"
  Conn1 : PMIOPort  Port=1  Side=Left
  Conn2 : PMIOPort  Port=2  Side=Right
  Conn3 : PMIOPort  Port=3  Side=Left
  Conn4 : PMIOPort  Port=4  Side=Right
  Out1 : Outport
  Out2 : Outport  Port=2
  Out3 : Outport  Port=3
  Out4 : Outport  Port=4
  Out5 : Outport  Port=5
  Out6 : Outport  Port=6
  Out7 : Outport  Port=7
  Out8 : Outport  Port=8
  Out9 : Outport  Port=9
  Out10 : Outport  Port=10
  wires:
  In8/1 -> Subsystem5/8(r_in)
  In3/1 -> Subsystem5/3(i_leak_in)
  In10/1 -> Subsystem5/10(l_in)
  In1/1 -> Subsystem5/1(v_r_in)
  In7/1 -> Subsystem5/7(c_in)
  In4/1 -> Subsystem5/4(p_chg_in)
  In5/1 -> Subsystem5/5(p_leak_in)
  In6/1 -> Subsystem5/6(i_in)
  In9/1 -> Subsystem5/9(r_leak_in)
  In2/1 -> Subsystem5/2(v_cap_in)
  Subsystem5/1(v_r_out) -> Subsystem1/1(v_r_in)
  Subsystem5/2(v_cap_out) -> Subsystem1/2(v_cap_in)
  Subsystem5/3(i_leak_out) -> Subsystem1/3(i_leak_in)
  Subsystem5/4(p_chg_out) -> Subsystem1/4(p_chg_in)
  Subsystem5/5(p_leak_out) -> Subsystem1/5(p_leak_in)
  Subsystem5/6(i_out) -> Subsystem1/6(i_in)
  Subsystem5/7(c_out) -> Subsystem1/7(c_in)
  Subsystem5/8(r_out) -> Subsystem1/8(r_in)
  Subsystem5/9(r_leak_out) -> Subsystem1/9(r_leak_in)
  Subsystem5/10(l_out) -> Subsystem1/10(l_in)
  Subsystem1/1(v_r_out) -> Subsystem2/1(v_r_in)
  Subsystem1/2(v_cap_out) -> Subsystem2/2(v_cap_in)
  Subsystem1/3(i_leak_out) -> Subsystem2/3(i_leak_in)
  Subsystem1/4(p_chg_out) -> Subsystem2/4(p_chg_in)
  Subsystem1/5(p_leak_out) -> Subsystem2/5(p_leak_in)
  Subsystem1/6(i_out) -> Subsystem2/6(i_in)
  Subsystem1/7(c_out) -> Subsystem2/7(c_in)
  Subsystem1/8(r_out) -> Subsystem2/8(r_in)
  Subsystem1/9(r_leak_out) -> Subsystem2/9(r_leak_in)
  Subsystem1/10(l_out) -> Subsystem2/10(l_in)
  Subsystem2/1(v_r_out) -> Subsystem3/1(v_r_in)
  Subsystem3/1(v_r_out) -> Out1/1
  Subsystem2/2(v_cap_out) -> Subsystem3/2(v_cap_in)
  Subsystem2/3(i_leak_out) -> Subsystem3/3(i_leak_in)
  Subsystem2/4(p_chg_out) -> Subsystem3/4(p_chg_in)
  Subsystem2/5(p_leak_out) -> Subsystem3/5(p_leak_in)
  Subsystem2/6(i_out) -> Subsystem3/6(i_in)
  Subsystem2/7(c_out) -> Subsystem3/7(c_in)
  Subsystem2/8(r_out) -> Subsystem3/8(r_in)
  Subsystem2/9(r_leak_out) -> Subsystem3/9(r_leak_in)
  Subsystem2/10(l_out) -> Subsystem3/10(l_in)
  Subsystem3/2(v_cap_out) -> Out2/1
  Subsystem3/3(i_leak_out) -> Out3/1
  Subsystem3/4(p_chg_out) -> Out4/1
  Subsystem3/5(p_leak_out) -> Out5/1
  Subsystem3/6(i_out) -> Out6/1
  Subsystem3/7(c_out) -> Out7/1
  Subsystem3/8(r_out) -> Out8/1
  Subsystem3/9(r_leak_out) -> Out9/1
  Subsystem3/10(l_out) -> Out10/1
  connections:
  Subsystem5/LConn2 -- Conn3/RConn1
  Subsystem5/LConn1 -- Conn1/RConn1
  Subsystem1/LConn1 -- Subsystem5/RConn1
  Subsystem1/LConn2 -- Subsystem5/RConn2
  Subsystem2/LConn1 -- Subsystem1/RConn1
  Subsystem2/LConn2 -- Subsystem1/RConn2
  Subsystem3/LConn1 -- Subsystem2/RConn1
  Subsystem3/LConn2 -- Subsystem2/RConn2
  Subsystem3/RConn1 -- Conn2/RConn1
  Subsystem3/RConn2 -- Conn4/RConn1

== system cap_eq_circuit_pascal5_single_shot_stack/Eq Circuit Network/Subsystem1 ==
  In1 : Inport
  In2 : Inport  Port=2
  In3 : Inport  Port=3
  In4 : Inport  Port=4
  In5 : Inport  Port=5
  In6 : Inport  Port=6
  In7 : Inport  Port=7
  In8 : Inport  Port=8
  In9 : Inport  Port=9
  In10 : Inport  Port=10
  Subsystem1 : Subsystem  mask{c=c, r_esr=r_esr, r_leak=r_leak, v_init=v_init}
      mask prompts: c "Capacitance /F"; r_esr "Series resistance /ohm"; r_leak "Leakage resistance /ohm (inf for disabled)"; v_init "Initial capacitor voltage"
  Subsystem2 : Subsystem  mask{c=c, r_esr=r_esr, r_leak=r_leak, v_init=v_init}
      mask prompts: c "Capacitance /F"; r_esr "Series resistance /ohm"; r_leak "Leakage resistance /ohm (inf for disabled)"; v_init "Initial capacitor voltage"
  Subsystem3 : Subsystem  mask{c=c, r_esr=r_esr, r_leak=r_leak, v_init=v_init}
      mask prompts: c "Capacitance /F"; r_esr "Series resistance /ohm"; r_leak "Leakage resistance /ohm (inf for disabled)"; v_init "Initial capacitor voltage"
  Subsystem5 : Subsystem  mask{c=c, r_esr=r_esr, r_leak=r_leak, v_init=v_init}
      mask prompts: c "Capacitance /F"; r_esr "Series resistance /ohm"; r_leak "Leakage resistance /ohm (inf for disabled)"; v_init "Initial capacitor voltage"
  Conn1 : PMIOPort  Port=1  Side=Left
  Conn2 : PMIOPort  Port=2  Side=Right
  Conn3 : PMIOPort  Port=3  Side=Left
  Conn4 : PMIOPort  Port=4  Side=Right
  Out1 : Outport
  Out2 : Outport  Port=2
  Out3 : Outport  Port=3
  Out4 : Outport  Port=4
  Out5 : Outport  Port=5
  Out6 : Outport  Port=6
  Out7 : Outport  Port=7
  Out8 : Outport  Port=8
  Out9 : Outport  Port=9
  Out10 : Outport  Port=10
  wires:
  Subsystem3/10(l_out) -> Out10/1
  Subsystem3/9(r_leak_out) -> Out9/1
  Subsystem3/8(r_out) -> Out8/1
  Subsystem3/7(c_out) -> Out7/1
  Subsystem3/6(i_out) -> Out6/1
  Subsystem3/5(p_leak_out) -> Out5/1
  Subsystem3/4(p_chg_out) -> Out4/1
  Subsystem3/3(i_leak_out) -> Out3/1
  Subsystem3/2(v_cap_out) -> Out2/1
  Subsystem2/10(l_out) -> Subsystem3/10(l_in)
  Subsystem2/9(r_leak_out) -> Subsystem3/9(r_leak_in)
  Subsystem2/8(r_out) -> Subsystem3/8(r_in)
  Subsystem2/7(c_out) -> Subsystem3/7(c_in)
  Subsystem2/6(i_out) -> Subsystem3/6(i_in)
  Subsystem2/5(p_leak_out) -> Subsystem3/5(p_leak_in)
  Subsystem2/4(p_chg_out) -> Subsystem3/4(p_chg_in)
  Subsystem2/3(i_leak_out) -> Subsystem3/3(i_leak_in)
  Subsystem2/2(v_cap_out) -> Subsystem3/2(v_cap_in)
  Subsystem3/1(v_r_out) -> Out1/1
  Subsystem2/1(v_r_out) -> Subsystem3/1(v_r_in)
  Subsystem1/10(l_out) -> Subsystem2/10(l_in)
  Subsystem1/9(r_leak_out) -> Subsystem2/9(r_leak_in)
  Subsystem1/8(r_out) -> Subsystem2/8(r_in)
  Subsystem1/7(c_out) -> Subsystem2/7(c_in)
  Subsystem1/6(i_out) -> Subsystem2/6(i_in)
  Subsystem1/5(p_leak_out) -> Subsystem2/5(p_leak_in)
  Subsystem1/4(p_chg_out) -> Subsystem2/4(p_chg_in)
  Subsystem1/3(i_leak_out) -> Subsystem2/3(i_leak_in)
  Subsystem1/2(v_cap_out) -> Subsystem2/2(v_cap_in)
  Subsystem1/1(v_r_out) -> Subsystem2/1(v_r_in)
  Subsystem5/10(l_out) -> Subsystem1/10(l_in)
  Subsystem5/9(r_leak_out) -> Subsystem1/9(r_leak_in)
  Subsystem5/8(r_out) -> Subsystem1/8(r_in)
  Subsystem5/7(c_out) -> Subsystem1/7(c_in)
  Subsystem5/6(i_out) -> Subsystem1/6(i_in)
  Subsystem5/5(p_leak_out) -> Subsystem1/5(p_leak_in)
  Subsystem5/4(p_chg_out) -> Subsystem1/4(p_chg_in)
  Subsystem5/3(i_leak_out) -> Subsystem1/3(i_leak_in)
  Subsystem5/2(v_cap_out) -> Subsystem1/2(v_cap_in)
  Subsystem5/1(v_r_out) -> Subsystem1/1(v_r_in)
  In2/1 -> Subsystem5/2(v_cap_in)
  In9/1 -> Subsystem5/9(r_leak_in)
  In6/1 -> Subsystem5/6(i_in)
  In5/1 -> Subsystem5/5(p_leak_in)
  In4/1 -> Subsystem5/4(p_chg_in)
  In7/1 -> Subsystem5/7(c_in)
  In1/1 -> Subsystem5/1(v_r_in)
  In10/1 -> Subsystem5/10(l_in)
  In3/1 -> Subsystem5/3(i_leak_in)
  In8/1 -> Subsystem5/8(r_in)
  connections:
  Subsystem3/RConn2 -- Conn4/RConn1
  Subsystem3/RConn1 -- Conn2/RConn1
  Subsystem3/LConn2 -- Subsystem2/RConn2
  Subsystem3/LConn1 -- Subsystem2/RConn1
  Subsystem2/LConn2 -- Subsystem1/RConn2
  Subsystem2/LConn1 -- Subsystem1/RConn1
  Subsystem1/LConn2 -- Subsystem5/RConn2
  Subsystem1/LConn1 -- Subsystem5/RConn1
  Subsystem5/LConn1 -- Conn1/RConn1
  Subsystem5/LConn2 -- Conn3/RConn1

== system cap_eq_circuit_pascal5_single_shot_stack/Eq Circuit Network/Subsystem2 ==
  In1 : Inport
  In2 : Inport  Port=2
  In3 : Inport  Port=3
  In4 : Inport  Port=4
  In5 : Inport  Port=5
  In6 : Inport  Port=6
  In7 : Inport  Port=7
  In8 : Inport  Port=8
  In9 : Inport  Port=9
  In10 : Inport  Port=10
  Subsystem1 : Subsystem  mask{c=c, r_esr=r_esr, r_leak=r_leak, v_init=v_init}
      mask prompts: c "Capacitance /F"; r_esr "Series resistance /ohm"; r_leak "Leakage resistance /ohm (inf for disabled)"; v_init "Initial capacitor voltage"
  Subsystem2 : Subsystem  mask{c=c, r_esr=r_esr, r_leak=r_leak, v_init=v_init}
      mask prompts: c "Capacitance /F"; r_esr "Series resistance /ohm"; r_leak "Leakage resistance /ohm (inf for disabled)"; v_init "Initial capacitor voltage"
  Subsystem3 : Subsystem  mask{c=c, r_esr=r_esr, r_leak=r_leak, v_init=v_init}
      mask prompts: c "Capacitance /F"; r_esr "Series resistance /ohm"; r_leak "Leakage resistance /ohm (inf for disabled)"; v_init "Initial capacitor voltage"
  Subsystem4 : Subsystem  mask{c=c, r_esr=r_esr, r_leak=r_leak, v_init=v_init}
      mask prompts: c "Capacitance /F"; r_esr "Series resistance /ohm"; r_leak "Leakage resistance /ohm (inf for disabled)"; v_init "Initial capacitor voltage"
  Subsystem5 : Subsystem  mask{c=c, r_esr=r_esr, r_leak=r_leak, v_init=v_init}
      mask prompts: c "Capacitance /F"; r_esr "Series resistance /ohm"; r_leak "Leakage resistance /ohm (inf for disabled)"; v_init "Initial capacitor voltage"
  Subsystem6 : Subsystem  mask{c=c, r_esr=r_esr, r_leak=r_leak, v_init=v_init}
      mask prompts: c "Capacitance /F"; r_esr "Series resistance /ohm"; r_leak "Leakage resistance /ohm (inf for disabled)"; v_init "Initial capacitor voltage"
  Conn1 : PMIOPort  Port=1  Side=Left
  Conn2 : PMIOPort  Port=2  Side=Right
  Conn3 : PMIOPort  Port=3  Side=Left
  Conn4 : PMIOPort  Port=4  Side=Right
  Out1 : Outport
  Out2 : Outport  Port=2
  Out3 : Outport  Port=3
  Out4 : Outport  Port=4
  Out5 : Outport  Port=5
  Out6 : Outport  Port=6
  Out7 : Outport  Port=7
  Out8 : Outport  Port=8
  Out9 : Outport  Port=9
  Out10 : Outport  Port=10
  wires:
  In1/1 -> Subsystem5/1(v_r_in)
  In2/1 -> Subsystem5/2(v_cap_in)
  In3/1 -> Subsystem5/3(i_leak_in)
  In4/1 -> Subsystem5/4(p_chg_in)
  In5/1 -> Subsystem5/5(p_leak_in)
  In6/1 -> Subsystem5/6(i_in)
  In7/1 -> Subsystem5/7(c_in)
  In8/1 -> Subsystem5/8(r_in)
  In9/1 -> Subsystem5/9(r_leak_in)
  In10/1 -> Subsystem5/10(l_in)
  Subsystem5/1(v_r_out) -> Subsystem1/1(v_r_in)
  Subsystem5/2(v_cap_out) -> Subsystem1/2(v_cap_in)
  Subsystem5/3(i_leak_out) -> Subsystem1/3(i_leak_in)
  Subsystem5/4(p_chg_out) -> Subsystem1/4(p_chg_in)
  Subsystem5/5(p_leak_out) -> Subsystem1/5(p_leak_in)
  Subsystem5/6(i_out) -> Subsystem1/6(i_in)
  Subsystem5/7(c_out) -> Subsystem1/7(c_in)
  Subsystem5/8(r_out) -> Subsystem1/8(r_in)
  Subsystem5/9(r_leak_out) -> Subsystem1/9(r_leak_in)
  Subsystem5/10(l_out) -> Subsystem1/10(l_in)
  Subsystem1/1(v_r_out) -> Subsystem2/1(v_r_in)
  Subsystem1/2(v_cap_out) -> Subsystem2/2(v_cap_in)
  Subsystem1/3(i_leak_out) -> Subsystem2/3(i_leak_in)
  Subsystem1/4(p_chg_out) -> Subsystem2/4(p_chg_in)
  Subsystem1/5(p_leak_out) -> Subsystem2/5(p_leak_in)
  Subsystem1/6(i_out) -> Subsystem2/6(i_in)
  Subsystem1/7(c_out) -> Subsystem2/7(c_in)
  Subsystem1/8(r_out) -> Subsystem2/8(r_in)
  Subsystem1/9(r_leak_out) -> Subsystem2/9(r_leak_in)
  Subsystem1/10(l_out) -> Subsystem2/10(l_in)
  Subsystem2/1(v_r_out) -> Subsystem3/1(v_r_in)
  Subsystem2/2(v_cap_out) -> Subsystem3/2(v_cap_in)
  Subsystem2/3(i_leak_out) -> Subsystem3/3(i_leak_in)
  Subsystem2/4(p_chg_out) -> Subsystem3/4(p_chg_in)
  Subsystem2/5(p_leak_out) -> Subsystem3/5(p_leak_in)
  Subsystem2/6(i_out) -> Subsystem3/6(i_in)
  Subsystem2/7(c_out) -> Subsystem3/7(c_in)
  Subsystem2/8(r_out) -> Subsystem3/8(r_in)
  Subsystem2/9(r_leak_out) -> Subsystem3/9(r_leak_in)
  Subsystem2/10(l_out) -> Subsystem3/10(l_in)
  Subsystem3/1(v_r_out) -> Subsystem4/1(v_r_in)
  Subsystem3/2(v_cap_out) -> Subsystem4/2(v_cap_in)
  Subsystem3/3(i_leak_out) -> Subsystem4/3(i_leak_in)
  Subsystem3/4(p_chg_out) -> Subsystem4/4(p_chg_in)
  Subsystem3/5(p_leak_out) -> Subsystem4/5(p_leak_in)
  Subsystem3/6(i_out) -> Subsystem4/6(i_in)
  Subsystem3/7(c_out) -> Subsystem4/7(c_in)
  Subsystem3/8(r_out) -> Subsystem4/8(r_in)
  Subsystem3/9(r_leak_out) -> Subsystem4/9(r_leak_in)
  Subsystem3/10(l_out) -> Subsystem4/10(l_in)
  Subsystem4/1(v_r_out) -> Subsystem6/1(v_r_in)
  Subsystem4/2(v_cap_out) -> Subsystem6/2(v_cap_in)
  Subsystem4/3(i_leak_out) -> Subsystem6/3(i_leak_in)
  Subsystem4/4(p_chg_out) -> Subsystem6/4(p_chg_in)
  Subsystem4/5(p_leak_out) -> Subsystem6/5(p_leak_in)
  Subsystem4/6(i_out) -> Subsystem6/6(i_in)
  Subsystem4/7(c_out) -> Subsystem6/7(c_in)
  Subsystem4/8(r_out) -> Subsystem6/8(r_in)
  Subsystem4/9(r_leak_out) -> Subsystem6/9(r_leak_in)
  Subsystem4/10(l_out) -> Subsystem6/10(l_in)
  Subsystem6/1(v_r_out) -> Out1/1
  Subsystem6/2(v_cap_out) -> Out2/1
  Subsystem6/3(i_leak_out) -> Out3/1
  Subsystem6/4(p_chg_out) -> Out4/1
  Subsystem6/5(p_leak_out) -> Out5/1
  Subsystem6/6(i_out) -> Out6/1
  Subsystem6/7(c_out) -> Out7/1
  Subsystem6/8(r_out) -> Out8/1
  Subsystem6/9(r_leak_out) -> Out9/1
  Subsystem6/10(l_out) -> Out10/1
  connections:
  Conn1/RConn1 -- Subsystem5/LConn1
  Conn3/RConn1 -- Subsystem5/LConn2
  Subsystem1/LConn1 -- Subsystem5/RConn1
  Subsystem1/LConn2 -- Subsystem5/RConn2
  Subsystem2/LConn1 -- Subsystem1/RConn1
  Subsystem2/LConn2 -- Subsystem1/RConn2
  Subsystem3/LConn1 -- Subsystem2/RConn1
  Subsystem3/LConn2 -- Subsystem2/RConn2
  Subsystem4/LConn1 -- Subsystem3/RConn1
  Subsystem4/LConn2 -- Subsystem3/RConn2
  Subsystem6/LConn1 -- Subsystem4/RConn1
  Subsystem6/LConn2 -- Subsystem4/RConn2
  Subsystem6/RConn1 -- Conn2/RConn1
  Subsystem6/RConn2 -- Conn4/RConn1
